simulink model "AGTF30SysDyn_PExPIn"  (R2023b)
settings: Solver=ode4  StartTime=0.0  StopTime=MWS.In.tend  FixedStep=MWS.In.Ts  RelTol=1e-3  EnableMultiTasking=on
model workspace: external: MAT-File (data not in the file)
values from neighbouring files (symbols this model uses):
  MWS = setup_initialize(MWS,startPt,SSsolverSP)    [Setup_Simulation.m]    (also in run_AGTF30e_script.m = Setup_Simulation(inputMethod,MWS.In,filename,Mdl,SSsolverSP))
undefined symbols (not defined in the file or in its folder): DiscIntNeverNeededParam
libraries: simulink x32, Lib_Solve_ModelSource_TMATS x28, Lib_EMTAT x27, Lib_Cntrl_FirstOrderSensor_TMATS x19, Lib_Cntrl_FirstOrderActuator_TMATS x2, Lib_Cntrl_LimitSelect_TMATS x2, Lib_Solve_OuterLoopIntegrator_TMATS x2, Lib_Cntrl_CorrectedSpeed_TMATS x1, Lib_Solve_IterNRSolverJC_TMATS x1, slpidlib x1
(part 1 of 8)
settings Model: Creator=jwchapm2  LastModifiedBy=jlkratz
settings SolverCC: AlgebraicLoopSolver=TrustRegion
settings DataIOCC: LimitDataPoints=on  SaveFormat=Array  ReturnWorkspaceOutputs=off
settings OptimizationCC: LifeSpan=inf
settings DebuggingCC: UnconnectedInputMsg=warning  UnconnectedOutputMsg=warning  UnconnectedLineMsg=warning  SFUnexpectedBacktrackingDiag=warning  SFNoUnconditionalDefaultTransitionDiag=warning  SFExecutionAtInitializationDiag=none  ArithmeticOperatorsInVariantConditions=warning
settings HardwareCC: ProdBitPerPointer=32  ProdBitPerSizeT=32  ProdBitPerPtrDiffT=32  ProdLargestAtomicFloat=None  ProdIntDivRoundTo=Undefined  ProdEndianess=Unspecified  ProdWordSize=32  ProdHWDeviceType=32-bit Generic
settings ModelReferenceCC: EnableRefExpFcnMdlSchedulingChecks=on  PropagateSignalLabelsOutOfModel=off
settings SFSimCC: SimUseLocalCustomCode=off  CustomCodeUndefinedFunction=UseInterfaceOnly
settings RTWCC: RTWUseLocalCustomCode=off  DLArmComputeVersion=19.05
settings CodeAppCC: StateflowObjectComments=on
settings GRTTargetCC: TargetLangStandard=C89/C90 (ANSI)
settings ConfigComp: CovMetricSettings=dw  CovSaveCumulativeToWorkspaceVar=on  CovSaveSingleToWorkspaceVar=on  CovExternalEMLEnable=off

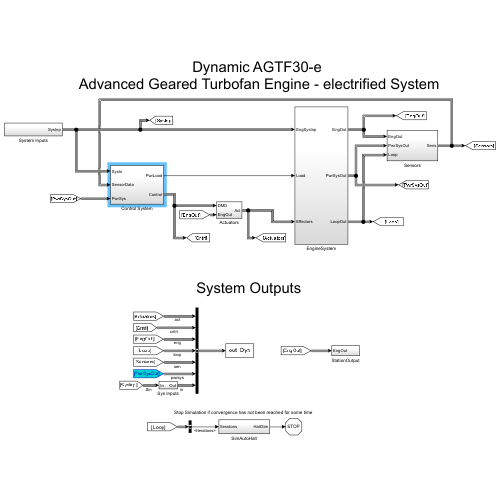
[thumbnail: Simulink's stored preview of the top-level diagram]
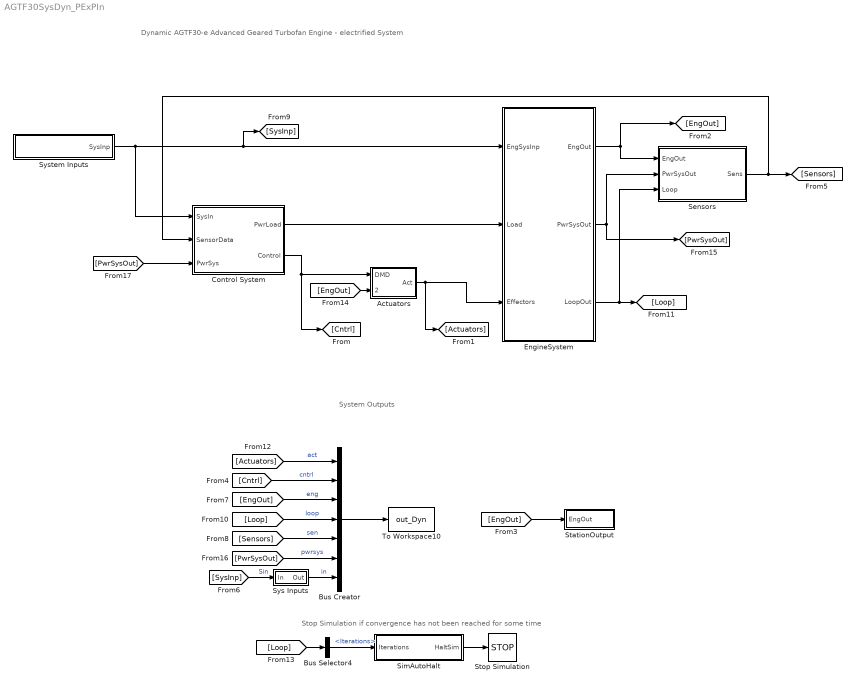
== system AGTF30SysDyn_PExPIn ==
  note: Stop Simulation if convergence has not been reached for some time
  note: Dynamic AGTF30-e
      | Advanced Geared Turbofan Engine - electrified System
  note: System Outputs
  Actuators : Subsystem
  Bus Creator : BusCreator  Inputs=7
  Bus Selector4 : BusSelector  OutputSignals=Solver.Iterations
  Control System : Subsystem
  EngineSystem : Subsystem
  Sensors : Subsystem
  SimAutoHalt : Subsystem
  StationOutput : Subsystem
  Stop Simulation : Stop
  Sys Inputs : Subsystem
  System Inputs : Subsystem
  To Workspace10 : ToWorkspace  VariableName=out_Dyn  SaveFormat=Timeseries  SampleTime=-1
  wires:
  Actuators/1(Act) -> [Actuators], EngineSystem/3(Effectors)
  Control System/2(Control) -> [Cntrl], Actuators/1(DMD)
  System Inputs/1(SysInp) -> Control System/1(SysIn), EngineSystem/1(EngSysInp), [SysInp]
  EngineSystem/1(EngOut) -> Sensors/1(EngOut), [EngOut]
  EngineSystem/3(LoopOut) -> Sensors/3(Loop), [Loop]
  [EngOut] -> StationOutput/1(EngOut)
  Bus Creator/1 -> To Workspace10/1
  [Loop] -> Bus Creator/4  "loop"
  [Sensors] -> Bus Creator/5  "sen"
  [EngOut] -> Bus Creator/3  "eng"
  Sys Inputs/1(Out) -> Bus Creator/7  "in"
  [Actuators] -> Bus Creator/1  "act"
  [Cntrl] -> Bus Creator/2  "cntrl"
  Sensors/1(Sens) -> Control System/2(SensorData), [Sensors]
  [Loop] -> Bus Selector4/1
  Bus Selector4/1 -> SimAutoHalt/1(Iterations)  "<Iterations>"
  SimAutoHalt/1(HaltSim) -> Stop Simulation/1
  [SysInp] -> Sys Inputs/1(In)  "Sin"
  EngineSystem/2(PwrSysOut) -> Sensors/2(PwrSysOut), [PwrSysOut]
  Control System/1(PwrLoad) -> EngineSystem/2(Load)
  [EngOut] -> Actuators/2(EngOut)
  [PwrSysOut] -> Bus Creator/6  "pwrsys"
  [PwrSysOut] -> Control System/3(PwrSys)

== system AGTF30SysDyn_PExPIn/Actuators ==
  DMD : Inport
  EngOut : Inport  Port=2
  Bus Creator : BusCreator  Inputs=9
  Bus Selector : BusSelector  OutputSignals=GBData.DEM.Nem,GBData.PGB.Nem
  Bus Selector1 : BusSelector  OutputSignals=Dmd.Wfdmd,Dmd.VBVdmd,Dmd.VAFNdmd,Dmd.TrqEMLdmd,Dmd.TrqEMHdmd,Dmd.TrqEMSdmd,Dmd.TrqEMRdmd,Dmd.TrqEMCdmd,Dmd.TrqEMPdmd
  Carrier Electric Machine : Subsystem
  Demux : Demux  Outputs=2
  Demux1 : Demux
  FMV : Subsystem
  HPS Electric Machine : Subsystem
  LPS Electric Machine : Subsystem
  Planet Gear Electric Machine : Subsystem
  Ring Gear Electric Machine : Subsystem
  Sun Gear Electric Machine : Subsystem
  VAFN : Subsystem
  VBV : Subsystem
  Act : Outport
  wires:
  DMD/1 -> Bus Selector1/1
  Bus Creator/1 -> Act/1  "Actuator"
  Bus Selector1/3 -> VAFN/1(VAFNdmd)  "<VAFNdmd>"
  Bus Selector1/2 -> VBV/1(VBVdmd)  "<VBVdmd>"
  VBV/1(VBVact) -> Bus Creator/2  "VBVact"
  VAFN/1(VAFNact) -> Bus Creator/3  "VAFNact"
  Bus Selector1/1 -> FMV/1(Wfdmd)  "<Wfdmd>"
  FMV/1(Wfact) -> Bus Creator/1  "Wfact"
  LPS Electric Machine/1(TrqEMLact) -> Bus Creator/4  "TrqEML"
  HPS Electric Machine/1(TrqEMHact) -> Bus Creator/5  "TrqEMH"
  Sun Gear Electric Machine/1(TrqEMSact) -> Bus Creator/6  "TrqEMS"
  Ring Gear Electric Machine/1(TrqEMRact) -> Bus Creator/7  "TrqEMR"
  Carrier Electric Machine/1(TrqEMCact) -> Bus Creator/8  "TrqEMC"
  Planet Gear Electric Machine/1(TrqEMPact) -> Bus Creator/9  "TrqEMP"
  Bus Selector1/4 -> LPS Electric Machine/1(TrqEMLdmd)  "<TrqEMLdmd>"
  Bus Selector1/5 -> HPS Electric Machine/1(TrqEMHdmd)  "<TrqEMHdmd>"
  Bus Selector1/6 -> Sun Gear Electric Machine/1(TrqEMSdmd)  "<TrqEMSdmd>"
  Bus Selector1/7 -> Ring Gear Electric Machine/1(TrqEMRdmd)  "<TrqEMRdmd>"
  Bus Selector1/8 -> Carrier Electric Machine/1(TrqEMCdmd)  "<TrqEMCdmd>"
  Bus Selector1/9 -> Planet Gear Electric Machine/1(TrqEMPdmd)  "<TrqEMPdmd>"
  EngOut/1 -> Bus Selector/1
  Bus Selector/1 -> Demux/1  "<Nem>"
  Bus Selector/2 -> Demux1/1  "<Nem>"
  Demux/1 -> LPS Electric Machine/2(NemL)
  Demux/2 -> HPS Electric Machine/2(NemH)
  Demux1/1 -> Sun Gear Electric Machine/2(NemS)
  Demux1/2 -> Ring Gear Electric Machine/2(NemR)
  Demux1/3 -> Carrier Electric Machine/2(NemC)
  Demux1/4 -> Planet Gear Electric Machine/2(NemP)

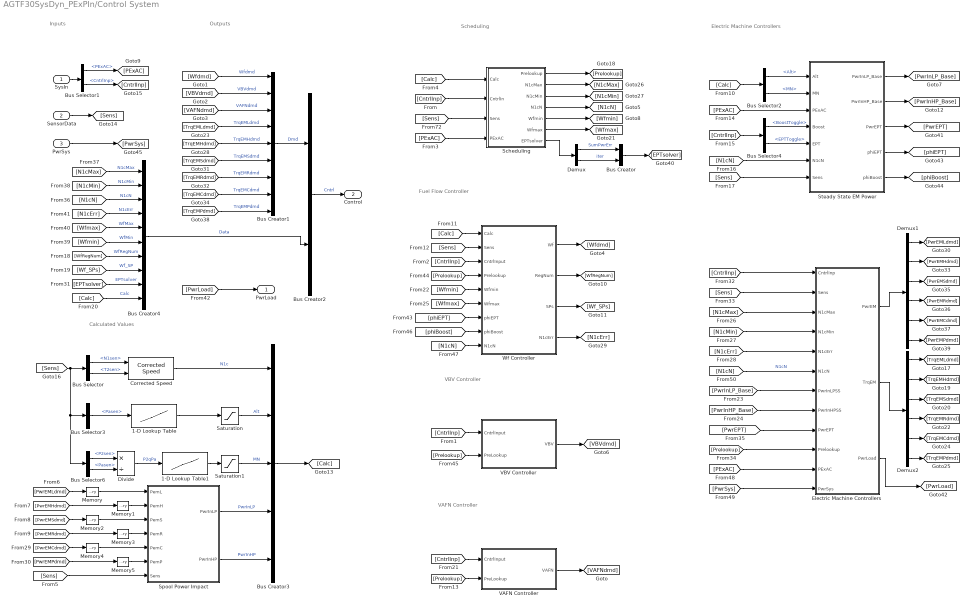
== system AGTF30SysDyn_PExPIn/Control System ==
  note: Inputs
  note: Calculated Values
  note: Outputs
  note: Fuel Flow Controller
  note: VBV Controller
  note: Scheduling
  note: VAFN Controller
  note: Electric Machine Controllers
  SysIn : Inport
  SensorData : Inport  Port=2
  PwrSys : Inport  Port=3
  1-D Lookup Table : Lookup_n-D  NumberOfTableDimensions=1  BreakpointsForDimension1=MWS.Cntrl.AltCalc_PaVec  Table=MWS.Cntrl.AltCalc_AltVec  InternalRulePriority=Speed  RndMeth=Simplest
  1-D Lookup Table1 : Lookup_n-D  NumberOfTableDimensions=1  BreakpointsForDimension1=MWS.Cntrl.MNCalc_P2qPa  Table=MWS.Cntrl.MNCalc_MNVec  InternalRulePriority=Speed  RndMeth=Simplest
  Bus Creator : BusCreator  Inputs=2
  Bus Creator1 : BusCreator  Inputs=9
  Bus Creator2 : BusCreator  Inputs=2
  Bus Creator3 : BusCreator  Inputs=5
  Bus Creator4 : BusCreator  Inputs=10
  Bus Selector : BusSelector  OutputSignals=N.N1sen,T.T2sen
  Bus Selector1 : BusSelector  OutputSignals=EngInp.PExAC,CntrlInp
  Bus Selector2 : BusSelector  OutputSignals=Alt,MN
  Bus Selector3 : BusSelector  OutputSignals=P.Pasen
  Bus Selector4 : BusSelector  OutputSignals=PilotCmd.BoostToggle,PilotCmd.EPTToggle
  Bus Selector6 : BusSelector  OutputSignals=P.P2sen,P.Pasen
  Corrected Speed : Lib_Cntrl_CorrectedSpeed_TMATS/Corrected Speed  C_TSTD_M=518.67
  Demux : Demux  Outputs=2
  Demux1 : Demux  Outputs=6
  Demux2 : Demux  Outputs=6
  Divide : Product  Inputs=*/
  Electric Machine Controllers : Subsystem
  Memory : Memory  InitialCondition=MWS.Init.IC.PwrEML
  Memory1 : Memory  InitialCondition=MWS.Init.IC.PwrEMH
  Memory2 : Memory  InitialCondition=MWS.Init.IC.PwrEMS
  Memory3 : Memory  InitialCondition=MWS.Init.IC.PwrEMR
  Memory4 : Memory  InitialCondition=MWS.Init.IC.PwrEMC
  Memory5 : Memory  InitialCondition=MWS.Init.IC.PwrEMP
  Saturation : Saturate  UpperLimit=MWS.Cntrl.AltCalc_Altmax  LowerLimit=MWS.Cntrl.AltCalc_Altmin
  Saturation1 : Saturate  UpperLimit=MWS.Cntrl.MNCalc_MNmax  LowerLimit=MWS.Cntrl.MNCalc_MNmin
  Scheduling : Subsystem
  Spool Power Impact : Subsystem
  Steady State EM Power : Subsystem
  VAFN Controller : Subsystem
  VBV Controller : Subsystem
  Wf Controller : Subsystem
  PwrLoad : Outport
  Control : Outport  Port=2
  wires:
  [Wfdmd] -> Bus Creator1/1  "Wfdmd"
  [VBVdmd] -> Bus Creator1/2  "VBVdmd"
  [VAFNdmd] -> Bus Creator1/3  "VAFNdmd"
  SensorData/1 -> [Sens]
  Bus Selector/1 -> Corrected Speed/1  "<N1sen>"
  Corrected Speed/1 -> Bus Creator3/1  "N1c"
  Bus Selector/2 -> Corrected Speed/2  "<T2sen>"
  1-D Lookup Table/1 -> Saturation/1
  [Sens] -> Bus Selector6/1, Bus Selector3/1, Bus Selector/1
  Bus Selector3/1 -> 1-D Lookup Table/1  "<Pasen>"
  Bus Selector6/1 -> Divide/1  "<P2sen>"
  Bus Selector6/2 -> Divide/2  "<Pasen>"
  Divide/1 -> 1-D Lookup Table1/1  "P2qPa"
  1-D Lookup Table1/1 -> Saturation1/1
  Saturation/1 -> Bus Creator3/2  "Alt"
  Saturation1/1 -> Bus Creator3/3  "MN"
  Bus Creator2/1 -> Control/1  "Cntrl"
  [TrqEMLdmd] -> Bus Creator1/4  "TrqEMLdmd"
  [TrqEMHdmd] -> Bus Creator1/5  "TrqEMHdmd"
  [TrqEMSdmd] -> Bus Creator1/6  "TrqEMSdmd"
  [TrqEMRdmd] -> Bus Creator1/7  "TrqEMRdmd"
  [TrqEMCdmd] -> Bus Creator1/8  "TrqEMCdmd"
  [TrqEMPdmd] -> Bus Creator1/9  "TrqEMPdmd"
  Bus Creator1/1 -> Bus Creator2/1  "Dmd"
  [Wfmax] -> Wf Controller/6(Wfmax)
  [Calc] -> Wf Controller/1(Calc)
  [Wfmin] -> Wf Controller/5(Wfmin)
  [Sens] -> Wf Controller/2(Sens)
  Wf Controller/1(Wf) -> [Wfdmd]
  [CntrlInp] -> Wf Controller/3(CntrlInput)
  Wf Controller/2(RegNum) -> [WfRegNum]
  Wf Controller/3(SPs) -> [Wf_SPs]
  [Prelookup] -> Wf Controller/4(Prelookup)
  [Prelookup] -> VBV Controller/2(PreLookup)
  VBV Controller/1(VBV) -> [VBVdmd]
  Scheduling/5(Wfmin) -> [Wfmin]
  Scheduling/4(N1cN) -> [N1cN]
  Scheduling/6(Wfmax) -> [Wfmax]
  Scheduling/1(Prelookup) -> [Prelookup]
  [CntrlInp] -> Scheduling/2(CntrlIn)
  [Sens] -> Scheduling/3(Sens)
  [Prelookup] -> VAFN Controller/2(PreLookup)
  VAFN Controller/1(VAFN) -> [VAFNdmd]
  SysIn/1 -> Bus Selector1/1
  Bus Selector1/2 -> [CntrlInp]  "<CntrlInp>"
  Bus Selector1/1 -> [PExAC]  "<PExAC>"
  Bus Creator3/1 -> [Calc]
  [Calc] -> Scheduling/1(Calc)
  Spool Power Impact/1(PwrInLP) -> Bus Creator3/4  "PwrInLP"
  Spool Power Impact/2(PwrInHP) -> Bus Creator3/5  "PwrInHP"
  [PExAC] -> Scheduling/4(PExAC)
  [PwrEMSdmd] -> Memory2/1
  [PwrEMRdmd] -> Memory3/1
  [PwrEMCdmd] -> Memory4/1
  [PwrEMPdmd] -> Memory5/1
  [PwrEMHdmd] -> Memory1/1
  [PwrEMLdmd] -> Memory/1
  [Sens] -> Spool Power Impact/7(Sens)
  Memory/1 -> Spool Power Impact/1(PemL)
  Memory1/1 -> Spool Power Impact/2(PemH)
  Memory2/1 -> Spool Power Impact/3(PemS)
  Memory3/1 -> Spool Power Impact/4(PemR)
  Memory4/1 -> Spool Power Impact/5(PemC)
  Memory5/1 -> Spool Power Impact/6(PemP)
  [CntrlInp] -> VAFN Controller/1(CntrlInput)
  [CntrlInp] -> VBV Controller/1(CntrlInput)
  Steady State EM Power/1(PwrInLP_Base) -> [PwrInLP_Base]
  Steady State EM Power/2(PwrInHP_Base) -> [PwrInHP_Base]
  [Calc] -> Bus Selector2/1
  Bus Selector2/1 -> Steady State EM Power/1(Alt)  "<Alt>"
  Bus Selector2/2 -> Steady State EM Power/2(MN)  "<MN>"
  [PExAC] -> Steady State EM Power/3(PExAC)
  [CntrlInp] -> Bus Selector4/1
  Bus Selector4/1 -> Steady State EM Power/4(Boost)  "<BoostToggle>"
  Bus Selector4/2 -> Steady State EM Power/5(EPT)  "<EPTToggle>"
  [N1cN] -> Steady State EM Power/6(N1cN)
  [Sens] -> Steady State EM Power/7(Sens)
  Scheduling/2(N1cMax) -> [N1cMax]
  Scheduling/3(N1cMin) -> [N1cMin]
  Wf Controller/4(N1cErr) -> [N1cErr]
  Scheduling/7(EPTsolver) -> Demux/1
  Demux/1 -> Bus Creator/1  "SumPwrErr"
  Demux/2 -> Bus Creator/2  "iter"
  Bus Creator/1 -> [EPTsolver]
  [PwrInHP_Base] -> Electric Machine Controllers/8(PwrInHPSS)
  [CntrlInp] -> Electric Machine Controllers/1(CntrlInp)
  [PwrInLP_Base] -> Electric Machine Controllers/7(PwrInLPSS)
  [N1cMax] -> Electric Machine Controllers/3(N1cMax)
  [N1cMin] -> Electric Machine Controllers/4(N1cMin)
  [N1cErr] -> Electric Machine Controllers/5(N1cErr)
  Demux1/1 -> [PwrEMLdmd]
  Demux1/2 -> [PwrEMHdmd]
  Demux1/3 -> [PwrEMSdmd]
  Demux1/4 -> [PwrEMRdmd]
  Demux1/5 -> [PwrEMCdmd]
  Demux1/6 -> [PwrEMPdmd]
  Demux2/1 -> [TrqEMLdmd]
  Demux2/2 -> [TrqEMHdmd]
  Demux2/3 -> [TrqEMSdmd]
  Demux2/4 -> [TrqEMRdmd]
  Demux2/5 -> [TrqEMCdmd]
  Demux2/6 -> [TrqEMPdmd]
  [Sens] -> Electric Machine Controllers/2(Sens)
  [Prelookup] -> Electric Machine Controllers/10(Prelookup)
  Electric Machine Controllers/1(PwrEM) -> Demux1/1
  Electric Machine Controllers/2(TrqEM) -> Demux2/1
  Steady State EM Power/3(PwrEPT) -> [PwrEPT]
  [PwrEPT] -> Electric Machine Controllers/9(PwrEPT)
  [EPTsolver] -> Bus Creator4/9  "EPTsolver"
  [Wf_SPs] -> Bus Creator4/8  "Wf_SP"
  [WfRegNum] -> Bus Creator4/7  "WfRegNum"
  [Wfmin] -> Bus Creator4/6  "WfMin"
  [Wfmax] -> Bus Creator4/5  "WfMax"
  [N1cErr] -> Bus Creator4/4  "N1cErr"
  [N1cN] -> Bus Creator4/3  "N1cN"
  [N1cMin] -> Bus Creator4/2  "N1cMin"
  [N1cMax] -> Bus Creator4/1  "N1cMax"
  [Calc] -> Bus Creator4/10  "Calc"
  Bus Creator4/1 -> Bus Creator2/2  "Data"
  [PwrLoad] -> PwrLoad/1
  Steady State EM Power/4(phiEPT) -> [phiEPT]
  Steady State EM Power/5(phiBoost) -> [phiBoost]
  [phiEPT] -> Wf Controller/7(phiEPT)
  [phiBoost] -> Wf Controller/8(phiBoost)
  [N1cN] -> Wf Controller/9(N1cN)
  [PwrSys] -> Electric Machine Controllers/12(PwrSys)
  PwrSys/1 -> [PwrSys]
  Electric Machine Controllers/3(PwrLoad) -> [PwrLoad]
  [PExAC] -> Electric Machine Controllers/11(PExAC)
  [N1cN] -> Electric Machine Controllers/6(N1cN)  "N1cN"

== system AGTF30SysDyn_PExPIn/EngineSystem ==
  note: Shaft Integrators
  note: Engine State
      | Integration Loop
  note: Engine Data Output
  note: Power System Data Output
  EngSysInp : Inport
  Load : Inport  Port=2
  Effectors : Inport  Port=3
  Bus Creator : BusCreator  Inputs=5
  EngineDW : Subsystem
  HP speed integrator : Lib_Solve_OuterLoopIntegrator_TMATS/OuterLoop integrator  OL_IC_M=MWS.Init.IC.N3
  LP shaft speed integrator : Lib_Solve_OuterLoopIntegrator_TMATS/OuterLoop integrator  OL_IC_M=MWS.Init.IC.N2
  Power System : Subsystem
  EngOut : Outport
  PwrSysOut : Outport  Port=2
  LoopOut : Outport  Port=3
  wires:
  EngSysInp/1 -> EngineDW/1(EngSysInp)
  LP shaft speed integrator/1 -> [N2], EngineDW/3(N2)  "N2int"
  Effectors/1 -> Power System/3(TrqEM), EngineDW/2(Effectors)
  EngineDW/3(N2dot) -> LP shaft speed integrator/1, [N2dot]  "N2dot"
  EngineDW/2(Solver) -> Bus Creator/1  "Solver"
  EngineDW/1(EngOut) -> [EngOut], EngOut/1
  EngineDW/4(N3dot) -> HP speed integrator/1, [N3dot]  "N3dot"
  HP speed integrator/1 -> [N3], EngineDW/4(N3)  "N3int"
  Bus Creator/1 -> LoopOut/1  "Loop"
  [N3dot] -> Bus Creator/2
  [N2dot] -> Bus Creator/3
  [N2] -> Bus Creator/4
  [N3] -> Bus Creator/5
  [EngOut] -> Power System/2(Nem)
  Power System/1(PwrSysOut) -> PwrSysOut/1
  Load/1 -> Power System/1(Load [hp])

== system AGTF30SysDyn_PExPIn/Sensors ==
  note: Pressure Sensors
  note: Temperature Sensors
  note: Speed Sensors
  EngOut : Inport
  PwrSysOut : Inport  Port=2
  Loop : Inport  Port=3
  Bus Creator : BusCreator  Inputs=4
  Bus Creator1 : BusCreator  Inputs=4
  Bus Creator2 : BusCreator  Inputs=5
  Bus Creator3 : BusCreator  Inputs=9
  Bus Selector : BusSelector  OutputSignals=Amb.Pa,S2.Pt,S25.Pt,S36.Ps,S5.Pt
  Bus Selector1 : BusSelector  OutputSignals=S2.Tt,S36.Tt,S4.Tt,S45.Tt
  Bus Selector2 : BusSelector  OutputSignals=N2int,N3int
  Bus Selector3 : BusSelector  OutputSignals=GBData.DEM.Nem,GBData.PGB.Nem
  Bus Selector4 : BusSelector  OutputSignals=SOC
  Demux : Demux  Outputs=2
  Demux1 : Demux
  Gain : Gain  Gain=1/MWS.GearBox.GearRatio
  N1 sensor : Lib_Cntrl_FirstOrderSensor_TMATS/1st order  Sensor  IC_M=MWS.Init.IC.N1  Sen_Max_M=MWS.Sensor.N1.Max  Sen_Min_M=MWS.Sensor.N1.Min  Gain_M=1  Tau_M=MWS.Sensor.N1.Tau  GN_EN_M=off  GN_NST_M=MWS.In.Ts  GN_C_M=1  GN_MinNoise_M=0.3  F_Gain_M=1  F_Drift_M=0
  N2 sensor : Lib_Cntrl_FirstOrderSensor_TMATS/1st order  Sensor  IC_M=MWS.Init.IC.N2  Sen_Max_M=MWS.Sensor.N2.Max  Sen_Min_M=MWS.Sensor.N2.Min  Gain_M=1  Tau_M=MWS.Sensor.N2.Tau  GN_EN_M=off  GN_NST_M=MWS.In.Ts  GN_C_M=1  GN_MinNoise_M=0.3  F_Gain_M=1  F_Drift_M=0
  N3 sensor : Lib_Cntrl_FirstOrderSensor_TMATS/1st order  Sensor  IC_M=MWS.Init.IC.N3  Sen_Max_M=MWS.Sensor.N3.Max  Sen_Min_M=MWS.Sensor.N3.Min  Gain_M=1  Tau_M=MWS.Sensor.N3.Tau  GN_EN_M=off  GN_NST_M=MWS.In.Ts  GN_C_M=1  GN_MinNoise_M=0.3  F_Gain_M=1  F_Drift_M=0
  NemC sensor : Lib_Cntrl_FirstOrderSensor_TMATS/1st order  Sensor  IC_M=MWS.Init.IC.NemC  Sen_Max_M=MWS.Sensor.NemC.Max  Sen_Min_M=MWS.Sensor.NemC.Min  Gain_M=1  Tau_M=MWS.Sensor.NemC.Tau  GN_EN_M=off  GN_NST_M=MWS.In.Ts  GN_C_M=1  GN_MinNoise_M=0.3  F_Gain_M=1  F_Drift_M=0
  NemH sensor : Lib_Cntrl_FirstOrderSensor_TMATS/1st order  Sensor  IC_M=MWS.Init.IC.NemH  Sen_Max_M=MWS.Sensor.NemH.Max  Sen_Min_M=MWS.Sensor.NemH.Min  Gain_M=1  Tau_M=MWS.Sensor.NemH.Tau  GN_EN_M=off  GN_NST_M=MWS.In.Ts  GN_C_M=1  GN_MinNoise_M=0.3  F_Gain_M=1  F_Drift_M=0
  NemL sensor : Lib_Cntrl_FirstOrderSensor_TMATS/1st order  Sensor  IC_M=MWS.Init.IC.NemL  Sen_Max_M=MWS.Sensor.NemL.Max  Sen_Min_M=MWS.Sensor.NemL.Min  Gain_M=1  Tau_M=MWS.Sensor.NemL.Tau  GN_EN_M=off  GN_NST_M=MWS.In.Ts  GN_C_M=1  GN_MinNoise_M=0.3  F_Gain_M=1  F_Drift_M=0
  NemP sensor : Lib_Cntrl_FirstOrderSensor_TMATS/1st order  Sensor  IC_M=MWS.Init.IC.NemP  Sen_Max_M=MWS.Sensor.NemP.Max  Sen_Min_M=MWS.Sensor.NemP.Min  Gain_M=1  Tau_M=MWS.Sensor.NemP.Tau  GN_EN_M=off  GN_NST_M=MWS.In.Ts  GN_C_M=1  GN_MinNoise_M=0.3  F_Gain_M=1  F_Drift_M=0
  NemR sensor : Lib_Cntrl_FirstOrderSensor_TMATS/1st order  Sensor  IC_M=MWS.Init.IC.NemR  Sen_Max_M=MWS.Sensor.NemR.Max  Sen_Min_M=MWS.Sensor.NemR.Min  Gain_M=1  Tau_M=MWS.Sensor.NemR.Tau  GN_EN_M=off  GN_NST_M=MWS.In.Ts  GN_C_M=1  GN_MinNoise_M=0.3  F_Gain_M=1  F_Drift_M=0
  NemS sensor : Lib_Cntrl_FirstOrderSensor_TMATS/1st order  Sensor  IC_M=MWS.Init.IC.NemS  Sen_Max_M=MWS.Sensor.NemS.Max  Sen_Min_M=MWS.Sensor.NemS.Min  Gain_M=1  Tau_M=MWS.Sensor.NemS.Tau  GN_EN_M=off  GN_NST_M=MWS.In.Ts  GN_C_M=1  GN_MinNoise_M=0.3  F_Gain_M=1  F_Drift_M=0
  Pamb sensor : Lib_Cntrl_FirstOrderSensor_TMATS/1st order  Sensor  IC_M=MWS.Init.IC.Pa  Sen_Max_M=MWS.Sensor.P2.Max  Sen_Min_M=MWS.Sensor.P2.Min  Gain_M=1  Tau_M=MWS.Sensor.P2.Tau  GN_EN_M=off  GN_NST_M=MWS.In.Ts  GN_C_M=1  GN_MinNoise_M=0.3  F_Gain_M=1  F_Drift_M=0
  Ps3 sensor : Lib_Cntrl_FirstOrderSensor_TMATS/1st order  Sensor  IC_M=MWS.Init.IC.Ps3  Sen_Max_M=MWS.Sensor.Ps3.Max  Sen_Min_M=MWS.Sensor.Ps3.Min  Gain_M=1  Tau_M=MWS.Sensor.Ps3.Tau  GN_EN_M=off  GN_NST_M=MWS.In.Ts  GN_C_M=1  GN_MinNoise_M=0.3  F_Gain_M=1  F_Drift_M=0
  Pt2 sensor : Lib_Cntrl_FirstOrderSensor_TMATS/1st order  Sensor  IC_M=MWS.Init.IC.P2  Sen_Max_M=MWS.Sensor.P2.Max  Sen_Min_M=MWS.Sensor.P2.Min  Gain_M=1  Tau_M=MWS.Sensor.P2.Tau  GN_EN_M=off  GN_NST_M=MWS.In.Ts  GN_C_M=1  GN_MinNoise_M=0.3  F_Gain_M=1  F_Drift_M=0
  Pt25 sensor : Lib_Cntrl_FirstOrderSensor_TMATS/1st order  Sensor  IC_M=MWS.Init.IC.P25  Sen_Max_M=MWS.Sensor.P25.Max  Sen_Min_M=MWS.Sensor.P25.Min  Gain_M=1  Tau_M=MWS.Sensor.P25.Tau  GN_EN_M=off  GN_NST_M=MWS.In.Ts  GN_C_M=1  GN_MinNoise_M=0.3  F_Gain_M=1  F_Drift_M=0
  Pt5 sensor : Lib_Cntrl_FirstOrderSensor_TMATS/1st order  Sensor  IC_M=MWS.Init.IC.P5  Sen_Max_M=MWS.Sensor.P5.Max  Sen_Min_M=MWS.Sensor.P5.Min  Gain_M=1  Tau_M=MWS.Sensor.P5.Tau  GN_EN_M=off  GN_NST_M=MWS.In.Ts  GN_C_M=1  GN_MinNoise_M=0.3  F_Gain_M=1  F_Drift_M=0
  SOC sensor : Lib_Cntrl_FirstOrderSensor_TMATS/1st order  Sensor  IC_M=MWS.Init.IC.SOC  Sen_Max_M=MWS.Sensor.SOC.Max  Sen_Min_M=MWS.Sensor.SOC.Min  Gain_M=1  Tau_M=MWS.Sensor.SOC.Tau  GN_EN_M=off  GN_NST_M=MWS.In.Ts  GN_C_M=1  GN_MinNoise_M=0.3  F_Gain_M=1  F_Drift_M=0
  T2 sensor : Lib_Cntrl_FirstOrderSensor_TMATS/1st order  Sensor  IC_M=MWS.Init.IC.T2  Sen_Max_M=MWS.Sensor.T2.Max  Sen_Min_M=MWS.Sensor.T2.Min  Gain_M=1  Tau_M=MWS.Sensor.T2.Tau  GN_EN_M=off  GN_NST_M=MWS.In.Ts  GN_C_M=1  GN_MinNoise_M=0.3  F_Gain_M=1  F_Drift_M=0
  T3 sensor : Lib_Cntrl_FirstOrderSensor_TMATS/1st order  Sensor  IC_M=MWS.Init.IC.T3  Sen_Max_M=MWS.Sensor.T3.Max  Sen_Min_M=MWS.Sensor.T3.Min  Gain_M=1  Tau_M=MWS.Sensor.T3.Tau  GN_EN_M=off  GN_NST_M=MWS.In.Ts  GN_C_M=1  GN_MinNoise_M=0.3  F_Gain_M=1  F_Drift_M=0
  T4 sensor : Lib_Cntrl_FirstOrderSensor_TMATS/1st order  Sensor  IC_M=MWS.Init.IC.T4  Sen_Max_M=MWS.Sensor.T4.Max  Sen_Min_M=MWS.Sensor.T4.Min  Gain_M=1  Tau_M=MWS.Sensor.T4.Tau  GN_EN_M=off  GN_NST_M=MWS.In.Ts  GN_C_M=1  GN_MinNoise_M=0.3  F_Gain_M=1  F_Drift_M=0
  T45 sensor : Lib_Cntrl_FirstOrderSensor_TMATS/1st order  Sensor  IC_M=MWS.Init.IC.T45  Sen_Max_M=MWS.Sensor.T45.Max  Sen_Min_M=MWS.Sensor.T45.Min  Gain_M=1  Tau_M=MWS.Sensor.T45.Tau  GN_EN_M=off  GN_NST_M=MWS.In.Ts  GN_C_M=1  GN_MinNoise_M=0.3  F_Gain_M=1  F_Drift_M=0
  Sens : Outport
  wires:
  Bus Creator/1 -> Sens/1  "Sensors"
  Bus Selector/2 -> Pt2 sensor/1  "<Pt>"
  Bus Creator2/1 -> Bus Creator/1  "P"
  Bus Creator1/1 -> Bus Creator/2  "T"
  Bus Selector1/1 -> T2 sensor/1  "<Tt>"
  Bus Creator3/1 -> Bus Creator/3  "N"
  Bus Selector/3 -> Pt25 sensor/1  "<Pt>"
  Bus Selector/5 -> Pt5 sensor/1  "<Pt>"
  Pt2 sensor/1 -> Bus Creator2/2  "P2sen"
  Pt25 sensor/1 -> Bus Creator2/3  "P25sen"
  Pt5 sensor/1 -> Bus Creator2/5  "P5sen"
  Bus Selector1/2 -> T3 sensor/1  "<Tt>"
  Bus Selector1/4 -> T45 sensor/1  "<Tt>"
  T2 sensor/1 -> Bus Creator1/1  "T2sen"
  T3 sensor/1 -> Bus Creator1/2  "T3sen"
  N1 sensor/1 -> Bus Creator3/1  "N1sen"
  Bus Selector/4 -> Ps3 sensor/1  "<Ps>"
  N3 sensor/1 -> Bus Creator3/3  "N3sen"
  Bus Selector/1 -> Pamb sensor/1  "<Pa>"
  Pamb sensor/1 -> Bus Creator2/1  "Pasen"
  N2 sensor/1 -> Bus Creator3/2  "N2sen"
  EngOut/1 -> Bus Selector3/1, Bus Selector/1, Bus Selector1/1
  Bus Selector2/2 -> N3 sensor/1  "<N3int>"
  Bus Selector2/1 -> N2 sensor/1, Gain/1  "<N2int>"
  Gain/1 -> N1 sensor/1
  Loop/1 -> Bus Selector2/1
  T45 sensor/1 -> Bus Creator1/4  "T45sen"
  Ps3 sensor/1 -> Bus Creator2/4  "Ps3sen"
  Bus Selector3/1 -> Demux/1  "<Nem>"
  Bus Selector3/2 -> Demux1/1  "<Nem>"
  NemL sensor/1 -> Bus Creator3/4  "NemLsen"
  NemH sensor/1 -> Bus Creator3/5  "NemHsen"
  Demux1/1 -> NemS sensor/1
  Demux1/2 -> NemR sensor/1
  Demux1/3 -> NemC sensor/1
  Demux1/4 -> NemP sensor/1
  Demux/1 -> NemL sensor/1
  Demux/2 -> NemH sensor/1
  NemS sensor/1 -> Bus Creator3/6  "NemSsen"
  NemR sensor/1 -> Bus Creator3/7  "NemRsen"
  NemC sensor/1 -> Bus Creator3/8  "NemCsen"
  NemP sensor/1 -> Bus Creator3/9  "NemPsen"
  Bus Selector1/3 -> T4 sensor/1  "<Tt>"
  T4 sensor/1 -> Bus Creator1/3  "T4sen"
  SOC sensor/1 -> Bus Creator/4  "SOC"
  PwrSysOut/1 -> Bus Selector4/1
  Bus Selector4/1 -> SOC sensor/1  "<SOC>"

== system AGTF30SysDyn_PExPIn/SimAutoHalt ==
  Iterations : Inport
  Compare To Constant : simulink/Logic and Bit Operations/Compare To Constant  relop=>=  const=MWS.Init.Max_IterDyn  OutDataTypeStr=boolean
  Compare To Constant1 : simulink/Logic and Bit Operations/Compare To Constant  relop=>=  const=MWS.Init.DynRunNonConv  OutDataTypeStr=boolean
  Constant : Constant
  Product : Product
  Sum : Sum  Inputs=|++
  Unit Delay : UnitDelay  SampleTime=-1  HasFrameUpgradeWarning=on
  HaltSim : Outport
  wires:
  Compare To Constant1/1 -> HaltSim/1
  Iterations/1 -> Compare To Constant/1
  Compare To Constant/1 -> Product/1
  Constant/1 -> Sum/1
  Sum/1 -> Unit Delay/1
  Unit Delay/1 -> Product/2
  Product/1 -> Sum/2, Compare To Constant1/1

== system AGTF30SysDyn_PExPIn/StationOutput ==
  EngOut : Inport
  Bus Selector1 : BusSelector  OutputSignals=Data.FAN_Data,Data.LPC_Data,Data.HPC_Data,Data.HPT_Data,Data.LPT_Data
  Bus Selector2 : BusSelector  OutputSignals=S0,S2,S21,S25,S36,S4,S45,S5,S17
  To Workspace : ToWorkspace  VariableName=out_S0  SaveFormat=Timeseries  SampleTime=-1
  To Workspace1 : ToWorkspace  VariableName=out_S2  SaveFormat=Timeseries  SampleTime=-1
  To Workspace10 : ToWorkspace  VariableName=out_HPCmp  SaveFormat=Timeseries  SampleTime=-1
  To Workspace11 : ToWorkspace  VariableName=out_HPTmp  SaveFormat=Timeseries  SampleTime=-1
  To Workspace12 : ToWorkspace  VariableName=out_LPTmp  SaveFormat=Timeseries  SampleTime=-1
  To Workspace13 : ToWorkspace  VariableName=out_S21  SaveFormat=Timeseries  SampleTime=-1
  To Workspace2 : ToWorkspace  VariableName=out_S25  SaveFormat=Timeseries  SampleTime=-1
  To Workspace3 : ToWorkspace  VariableName=out_S36  SaveFormat=Timeseries  SampleTime=-1
  To Workspace4 : ToWorkspace  VariableName=out_S4  SaveFormat=Timeseries  SampleTime=-1
  To Workspace5 : ToWorkspace  VariableName=out_S45  SaveFormat=Timeseries  SampleTime=-1
  To Workspace6 : ToWorkspace  VariableName=out_S5  SaveFormat=Timeseries  SampleTime=-1
  To Workspace7 : ToWorkspace  VariableName=out_S17  SaveFormat=Timeseries  SampleTime=-1
  To Workspace8 : ToWorkspace  VariableName=out_FANmp  SaveFormat=Timeseries  SampleTime=-1
  To Workspace9 : ToWorkspace  VariableName=out_LPCmp  SaveFormat=Timeseries  SampleTime=-1
  wires:
  Bus Selector2/3 -> To Workspace13/1  "<S21>"
  Bus Selector2/1 -> To Workspace/1  "<S0>"
  EngOut/1 -> Bus Selector1/1, Bus Selector2/1
  Bus Selector2/2 -> To Workspace1/1  "<S2>"
  Bus Selector2/4 -> To Workspace2/1  "<S25>"
  Bus Selector2/5 -> To Workspace3/1  "<S36>"
  Bus Selector2/6 -> To Workspace4/1  "<S4>"
  Bus Selector2/7 -> To Workspace5/1  "<S45>"
  Bus Selector2/8 -> To Workspace6/1  "<S5>"
  Bus Selector2/9 -> To Workspace7/1  "<S17>"
  Bus Selector1/1 -> To Workspace8/1  "<FAN_Data>"
  Bus Selector1/2 -> To Workspace9/1  "<LPC_Data>"
  Bus Selector1/3 -> To Workspace10/1  "<HPC_Data>"
  Bus Selector1/4 -> To Workspace11/1  "<HPT_Data>"
  Bus Selector1/5 -> To Workspace12/1  "<LPT_Data>"

== system AGTF30SysDyn_PExPIn/Sys Inputs ==
  In : Inport
  Bus Creator1 : BusCreator  Inputs=28
  Bus Selector : BusSelector  OutputSignals=EngInp.Alt,EngInp.dT,EngInp.MN,EngInp.PExAC,CntrlInp.PilotCmd.PLA,CntrlInp.PilotCmd.BoostToggle,CntrlInp.PilotCmd.EPTToggle,CntrlInp.PilotCmd.ChargingToggle,CntrlInp.ManualOp.N1cMan,CntrlInp.ManualOp.WfMan,CntrlInp.ManualOp.VBVMan,CntrlInp.ManualOp.VAFNMan,CntrlInp.ManualOp.PwrInLPNomMan,CntrlInp.ManualOp.PwrInLPOffNomMan,CntrlInp.ManualOp.PwrInHPNomMan,CntrlInp.ManualOp.PwrInHPOffNomMan,CntrlInp.ManualOp.PwrInLPEMNomMan,CntrlInp.ManualOp.PwrInLPEMOffNomMan,CntrlInp.ManualOp.PwrInHPEMNomMan,CntrlInp.ManualOp.PwrInHPEMOffNomMan,CntrlInp.ManualOp.PwrInSEMNomMan,CntrlInp.ManualOp.PwrInSEMOffNomMan,CntrlInp.ManualOp.PwrInREMNomMan,CntrlInp.ManualOp.PwrInREMOffNomMan,CntrlInp.ManualOp.PwrInCEMNomMan,CntrlInp.ManualOp.PwrInCEMOffNomMan,CntrlInp.ManualOp.PwrInPEMNomMan,CntrlInp.ManualOp.PwrInPEMOffNomMan
  Out : Outport
  wires:
  In/1 -> Bus Selector/1
  Bus Selector/4 -> Bus Creator1/4  "<PExAC>"
  Bus Selector/6 -> Bus Creator1/6  "<BoostToggle>"
  Bus Selector/7 -> Bus Creator1/7  "<EPTToggle>"
  Bus Selector/8 -> Bus Creator1/8  "<ChargingToggle>"
  Bus Selector/10 -> Bus Creator1/10  "<WfMan>"
  Bus Selector/13 -> Bus Creator1/13  "<PwrInLPNomMan>"
  Bus Selector/3 -> Bus Creator1/3  "<MN>"
  Bus Selector/5 -> Bus Creator1/5  "<PLA>"
  Bus Selector/1 -> Bus Creator1/1  "<Alt>"
  Bus Selector/12 -> Bus Creator1/12  "<VAFNMan>"
  Bus Selector/2 -> Bus Creator1/2  "<dT>"
  Bus Creator1/1 -> Out/1
  Bus Selector/14 -> Bus Creator1/14  "<PwrInLPOffNomMan>"
  Bus Selector/15 -> Bus Creator1/15  "<PwrInHPNomMan>"
  Bus Selector/16 -> Bus Creator1/16  "<PwrInHPOffNomMan>"
  Bus Selector/17 -> Bus Creator1/17  "<PwrInLPEMNomMan>"
  Bus Selector/18 -> Bus Creator1/18  "<PwrInLPEMOffNomMan>"
  Bus Selector/19 -> Bus Creator1/19  "<PwrInHPEMNomMan>"
  Bus Selector/20 -> Bus Creator1/20  "<PwrInHPEMOffNomMan>"
  Bus Selector/22 -> Bus Creator1/22  "<PwrInSEMOffNomMan>"
  Bus Selector/23 -> Bus Creator1/23  "<PwrInREMNomMan>"
  Bus Selector/24 -> Bus Creator1/24  "<PwrInREMOffNomMan>"
  Bus Selector/26 -> Bus Creator1/26  "<PwrInCEMOffNomMan>"
  Bus Selector/27 -> Bus Creator1/27  "<PwrInPEMNomMan>"
  Bus Selector/28 -> Bus Creator1/28  "<PwrInPEMOffNomMan>"
  Bus Selector/25 -> Bus Creator1/25  "<PwrInCEMNomMan>"
  Bus Selector/21 -> Bus Creator1/21  "<PwrInSEMNomMan>"
  Bus Selector/11 -> Bus Creator1/11  "<VBVMan>"
  Bus Selector/9 -> Bus Creator1/9  "<N1cMan>"

== system AGTF30SysDyn_PExPIn/System Inputs ==
  note: Engine Inputs
  note: Control System Inputs
  note: 40 - 80 angle
  Bus Creator : BusCreator  Inputs=4
  Bus Creator1 : BusCreator  Inputs=4
  Bus Creator2 : BusCreator  Inputs=2
  Bus Creator5 : BusCreator  Inputs=2
  Bus Creator6 : BusCreator  Inputs=40
  Constant1 : Constant  Value=MWS.In.WfManEn
  Constant10 : Constant  Value=MWS.In.PwrInHPEMOffNomManEn
  Constant11 : Constant  Value=MWS.In.PwrInLPEMOffNomManEn
  Constant12 : Constant  Value=MWS.In.PwrInLPEMNomManEn
  Constant13 : Constant  Value=MWS.In.PwrInSEMOffNomManEn
  Constant14 : Constant  Value=MWS.In.PwrInSEMNomManEn
  Constant15 : Constant  Value=MWS.In.PwrInREMOffNomManEn
  Constant16 : Constant  Value=MWS.In.PwrInREMNomManEn
  Constant17 : Constant  Value=MWS.In.PwrInCEMOffNomManEn
  Constant18 : Constant  Value=MWS.In.PwrInCEMNomManEn
  Constant19 : Constant  Value=MWS.In.PwrInPEMOffNomManEn
  Constant2 : Constant  Value=MWS.In.PwrInLPNomManEn
  Constant20 : Constant  Value=MWS.In.PwrInPEMNomManEn
  Constant3 : Constant  Value=MWS.In.VBVManEn
  Constant4 : Constant  Value=MWS.In.VAFNManEn
  Constant5 : Constant  Value=MWS.In.N1cManEn
  Constant6 : Constant  Value=MWS.In.PwrInHPNomManEn
  Constant7 : Constant  Value=MWS.In.PwrInLPOffNomManEn
  Constant8 : Constant  Value=MWS.In.PwrInHPOffNomManEn
  Constant9 : Constant  Value=MWS.In.PwrInHPEMNomManEn
  Model Source : Lib_Solve_ModelSource_TMATS/Model Source  T_vec_M=MWS.In.t_WfMan  input_array_M=MWS.In.WfMan
  Model Source1 : Lib_Solve_ModelSource_TMATS/Model Source  T_vec_M=MWS.In.t_Alt  input_array_M=MWS.In.Alt
  Model Source10 : Lib_Solve_ModelSource_TMATS/Model Source  T_vec_M=MWS.In.t_PwrInLPOffNomMan  input_array_M=MWS.In.PwrInLPOffNomMan
  Model Source11 : Lib_Solve_ModelSource_TMATS/Model Source  T_vec_M=MWS.In.t_PwrInHPOffNomMan  input_array_M=MWS.In.PwrInHPOffNomMan
  Model Source12 : Lib_Solve_ModelSource_TMATS/Model Source  T_vec_M=MWS.In.t_PwrInHPEMOffNomMan  input_array_M=MWS.In.PwrInHPEMOffNomMan
  Model Source13 : Lib_Solve_ModelSource_TMATS/Model Source  T_vec_M=MWS.In.t_PwrInHPEMNomMan  input_array_M=MWS.In.PwrInHPEMNomMan
  Model Source14 : Lib_Solve_ModelSource_TMATS/Model Source  T_vec_M=MWS.In.t_PwrInLPEMOffNomMan  input_array_M=MWS.In.PwrInLPEMOffNomMan
  Model Source15 : Lib_Solve_ModelSource_TMATS/Model Source  T_vec_M=MWS.In.t_PwrInLPEMNomMan  input_array_M=MWS.In.PwrInLPEMNomMan
  Model Source16 : Lib_Solve_ModelSource_TMATS/Model Source  T_vec_M=MWS.In.t_PwrInSEMOffNomMan  input_array_M=MWS.In.PwrInSEMOffNomMan
  Model Source17 : Lib_Solve_ModelSource_TMATS/Model Source  T_vec_M=MWS.In.t_PwrInSEMNomMan  input_array_M=MWS.In.PwrInSEMNomMan
  Model Source18 : Lib_Solve_ModelSource_TMATS/Model Source  T_vec_M=MWS.In.t_PwrInREMOffNomMan  input_array_M=MWS.In.PwrInREMOffNomMan
  Model Source19 : Lib_Solve_ModelSource_TMATS/Model Source  T_vec_M=MWS.In.t_PwrInREMNomMan  input_array_M=MWS.In.PwrInREMNomMan
  Model Source2 : Lib_Solve_ModelSource_TMATS/Model Source  T_vec_M=MWS.In.t_dTamb  input_array_M=MWS.In.dTamb
  Model Source20 : Lib_Solve_ModelSource_TMATS/Model Source  T_vec_M=MWS.In.t_PwrInCEMOffNomMan  input_array_M=MWS.In.PwrInCEMOffNomMan
  Model Source21 : Lib_Solve_ModelSource_TMATS/Model Source  T_vec_M=MWS.In.t_PwrInCEMNomMan  input_array_M=MWS.In.PwrInCEMNomMan
  Model Source22 : Lib_Solve_ModelSource_TMATS/Model Source  T_vec_M=MWS.In.t_PwrInPEMOffNomMan  input_array_M=MWS.In.PwrInPEMOffNomMan
  Model Source23 : Lib_Solve_ModelSource_TMATS/Model Source  T_vec_M=MWS.In.t_PwrInPEMNomMan  input_array_M=MWS.In.PwrInPEMNomMan
  Model Source24 : Lib_Solve_ModelSource_TMATS/Model Source  T_vec_M=MWS.In.t_Boost  input_array_M=MWS.In.Boost
  Model Source25 : Lib_Solve_ModelSource_TMATS/Model Source  T_vec_M=MWS.In.t_EPT  input_array_M=MWS.In.EPT
  Model Source26 : Lib_Solve_ModelSource_TMATS/Model Source  T_vec_M=MWS.In.t_PExAC  input_array_M=MWS.In.PExAC
  Model Source27 : Lib_Solve_ModelSource_TMATS/Model Source  T_vec_M=MWS.In.t_Charge  input_array_M=MWS.In.Charge
  Model Source3 : Lib_Solve_ModelSource_TMATS/Model Source  T_vec_M=MWS.In.t_MN  input_array_M=MWS.In.MN
  Model Source4 : Lib_Solve_ModelSource_TMATS/Model Source  T_vec_M=MWS.In.t_PLA  input_array_M=MWS.In.PLA
  Model Source5 : Lib_Solve_ModelSource_TMATS/Model Source  T_vec_M=MWS.In.t_PwrInLPNomMan  input_array_M=MWS.In.PwrInLPNomMan
  Model Source6 : Lib_Solve_ModelSource_TMATS/Model Source  T_vec_M=MWS.In.t_VBVMan  input_array_M=MWS.In.VBVMan
  Model Source7 : Lib_Solve_ModelSource_TMATS/Model Source  T_vec_M=MWS.In.t_VAFNMan  input_array_M=MWS.In.VAFNMan
  Model Source8 : Lib_Solve_ModelSource_TMATS/Model Source  T_vec_M=MWS.In.t_N1cMan  input_array_M=MWS.In.N1cMan
  Model Source9 : Lib_Solve_ModelSource_TMATS/Model Source  T_vec_M=MWS.In.t_PwrInHPNomMan  input_array_M=MWS.In.PwrInHPNomMan
  SysInp : Outport
  wires:
  Model Source1/1 -> Bus Creator/1  "Alt"
  Model Source2/1 -> Bus Creator/2  "dT"
  Model Source3/1 -> Bus Creator/3  "MN"
  Bus Creator/1 -> Bus Creator2/1  "EngInp"
  Bus Creator5/1 -> Bus Creator2/2  "CntrlInp"
  Bus Creator2/1 -> SysInp/1  "SysInp"
  Model Source6/1 -> Bus Creator6/5  "VBVMan"
  Model Source7/1 -> Bus Creator6/7  "VAFNMan"
  Model Source4/1 -> Bus Creator1/1  "PLA"
  Bus Creator6/1 -> Bus Creator5/2  "ManualOp"
  Model Source/1 -> Bus Creator6/1  "WfMan"
  Constant1/1 -> Bus Creator6/2  "WfManEn"
  Constant4/1 -> Bus Creator6/8  "VAFNManEn"
  Constant3/1 -> Bus Creator6/6  "VBVManEn"
  Model Source8/1 -> Bus Creator6/3  "N1cMan"
  Constant5/1 -> Bus Creator6/4  "N1cManEn"
  Model Source5/1 -> Bus Creator6/9  "PwrInLPNomMan"
  Constant2/1 -> Bus Creator6/10  "PwrInLPNomManEn"
  Model Source10/1 -> Bus Creator6/11  "PwrInLPOffNomMan"
  Constant7/1 -> Bus Creator6/12  "PwrInLPOffNomManEn"
  Model Source9/1 -> Bus Creator6/13  "PwrInHPNomMan"
  Constant6/1 -> Bus Creator6/14  "PwrInHPNomManEn"
  Model Source11/1 -> Bus Creator6/15  "PwrInHPOffNomMan"
  Constant8/1 -> Bus Creator6/16  "PwrInHPOffNomManEn"
  Model Source15/1 -> Bus Creator6/17  "PwrInLPEMNomMan"
  Constant12/1 -> Bus Creator6/18  "PwrInLPEMNomManEn"
  Model Source14/1 -> Bus Creator6/19  "PwrInLPEMOffNomMan"
  Constant11/1 -> Bus Creator6/20  "PwrInLPEMOffNomManEn"
  Model Source13/1 -> Bus Creator6/21  "PwrInHPEMNomMan"
  Constant9/1 -> Bus Creator6/22  "PwrInHPEMNomManEn"
  Model Source12/1 -> Bus Creator6/23  "PwrInHPEMOffNomMan"
  Constant10/1 -> Bus Creator6/24  "PwrInHPEMOffNomManEn"
  Model Source17/1 -> Bus Creator6/25  "PwrInSEMNomMan"
  Constant14/1 -> Bus Creator6/26  "PwrInSEMNomManEn"
  Model Source16/1 -> Bus Creator6/27  "PwrInSEMOffNomMan"
  Constant13/1 -> Bus Creator6/28  "PwrInSEMOffNomManEn"
  Model Source19/1 -> Bus Creator6/29  "PwrInREMNomMan"
  Constant16/1 -> Bus Creator6/30  "PwrInREMNomManEn"
  Model Source18/1 -> Bus Creator6/31  "PwrInREMOffNomMan"
  Constant15/1 -> Bus Creator6/32  "PwrInREMOffNomManEn"
  Model Source21/1 -> Bus Creator6/33  "PwrInCEMNomMan"
  Constant18/1 -> Bus Creator6/34  "PwrInCEMNomManEn"
  Model Source20/1 -> Bus Creator6/35  "PwrInCEMOffNomMan"
  Constant17/1 -> Bus Creator6/36  "PwrInCEMOffNomManEn"
  Model Source23/1 -> Bus Creator6/37  "PwrInPEMNomMan"
  Constant20/1 -> Bus Creator6/38  "PwrInPEMNomManEn"
  Model Source22/1 -> Bus Creator6/39  "PwrInPEMOffNomMan"
  Constant19/1 -> Bus Creator6/40  "PwrInPEMOffNomManEn"
  Bus Creator1/1 -> Bus Creator5/1  "PilotCmd"
  Model Source24/1 -> Bus Creator1/2  "BoostToggle"
  Model Source25/1 -> Bus Creator1/3  "EPTToggle"
  Model Source26/1 -> Bus Creator/4  "PExAC"
  Model Source27/1 -> Bus Creator1/4  "ChargingToggle"

== system AGTF30SysDyn_PExPIn/Actuators/Carrier Electric Machine ==
  TrqEMCdmd : Inport
  NemC : Inport  Port=2
  Abs : Abs  SaturateOnIntegerOverflow=off
  Abs1 : Abs  SaturateOnIntegerOverflow=off
  Constant : Constant  Value=MWS.PowerSystem.EMC.PMax
  Constant1 : Constant  Value=MWS.In.Ts
  Constant2 : Constant  Value=MWS.Act.EMC.RLmax
  Constant3 : Constant  Value=MWS.Act.EMC.RLmin
  Divide : Product  Inputs=**
  Low Spool Electric Machine Dynamics : StateSpace  A=MWS.Act.EMC.A  B=MWS.Act.EMC.B  C=MWS.Act.EMC.C  D=MWS.Act.EMC.D  InitialCondition=MWS.Init.IC.TrqEMC
  Memory3 : Memory  InitialCondition=MWS.Init.IC.TrqEMC
  Memory5 : Memory  InitialCondition=MWS.Init.IC.NemC
  Power [hp] to Torque [ft-lb] : Subsystem
  Rate Limit Enforcement : MATLAB Function  TreatAsAtomicUnit=on
  Relational Operator : RelationalOperator  Operator=<=  OutDataTypeStr=boolean  RndMeth=Simplest  InputSameDT=off
  Saturation1 : Saturate  UpperLimit=MWS.PowerSystem.EMC.TrqMax  LowerLimit=-MWS.PowerSystem.EMC.TrqMax  LinearizeAsGain=off
  Sign : Signum
  Switch : Switch  Criteria=u2 > Threshold  SaturateOnIntegerOverflow=off  InputSameDT=off
  TrqEMCact : Outport  VectorParamsAs1DForOutWhenUnconnected=off
  wires:
  Low Spool Electric Machine Dynamics/1 -> Saturation1/1
  Constant/1 -> Power [hp] to Torque [ft-lb]/2(P)
  Saturation1/1 -> Switch/3, Sign/1, Abs/1
  Power [hp] to Torque [ft-lb]/1(Trq) -> Abs1/1
  Abs/1 -> Relational Operator/2
  Relational Operator/1 -> Switch/2
  Divide/1 -> Switch/1
  Sign/1 -> Divide/2
  Constant1/1 -> Rate Limit Enforcement/5(dt)
  Constant2/1 -> Rate Limit Enforcement/4(Mdot_hi)
  Constant3/1 -> Rate Limit Enforcement/3(Mdot_low)
  Memory3/1 -> Rate Limit Enforcement/2(M_old)
  Switch/1 -> Rate Limit Enforcement/1(M_preRL)
  NemC/1 -> Memory5/1
  Memory5/1 -> Power [hp] to Torque [ft-lb]/1(N)
  Rate Limit Enforcement/1(M_act) -> TrqEMCact/1, Memory3/1
  TrqEMCdmd/1 -> Low Spool Electric Machine Dynamics/1
  Abs1/1 -> Divide/1, Relational Operator/1

== system AGTF30SysDyn_PExPIn/Actuators/FMV ==
  Wfdmd : Inport
  1st order Actuator : Lib_Cntrl_FirstOrderActuator_TMATS/1st order Actuator  Gain_M=MWS.Act.FMV.Gain  Tau_M=MWS.Act.FMV.Tau  IC_M=MWS.Init.IC.Wf  MaxSat_M=MWS.Act.FMV.max  MinSat_M=MWS.Act.FMV.min  deadband_M=0.0  rateLimit_M=MWS.Act.FMV.rateLimit
  Wf delay : TransportDelay  DelayTime=MWS.Act.FMV.TWf_dly  InitialOutput=MWS.Init.IC.Wf
  Wfact : Outport
  wires:
  Wf delay/1 -> Wfact/1  "Wfact"
  Wfdmd/1 -> 1st order Actuator/1
  1st order Actuator/1 -> Wf delay/1

== system AGTF30SysDyn_PExPIn/Actuators/HPS Electric Machine ==
  TrqEMHdmd : Inport
  NemH : Inport  Port=2
  Abs : Abs  SaturateOnIntegerOverflow=off
  Abs1 : Abs  SaturateOnIntegerOverflow=off
  Constant : Constant  Value=MWS.PowerSystem.EMH.PMax
  Constant1 : Constant  Value=MWS.In.Ts
  Constant2 : Constant  Value=MWS.Act.EMH.RLmax
  Constant3 : Constant  Value=MWS.Act.EMH.RLmin
  Divide : Product  Inputs=**
  Low Spool Electric Machine Dynamics : StateSpace  A=MWS.Act.EMH.A  B=MWS.Act.EMH.B  C=MWS.Act.EMH.C  D=MWS.Act.EMH.D  InitialCondition=MWS.Init.IC.TrqEMH
  Memory3 : Memory  InitialCondition=MWS.Init.IC.TrqEMH
  Memory5 : Memory  InitialCondition=MWS.Init.IC.NemH
  Power [hp] to Torque [ft-lb] : Subsystem
  Rate Limit Enforcement : MATLAB Function  TreatAsAtomicUnit=on
  Relational Operator : RelationalOperator  Operator=<=  OutDataTypeStr=boolean  RndMeth=Simplest  InputSameDT=off
  Saturation1 : Saturate  UpperLimit=MWS.PowerSystem.EMH.TrqMax  LowerLimit=-MWS.PowerSystem.EMH.TrqMax  LinearizeAsGain=off
  Sign : Signum
  Switch : Switch  Criteria=u2 > Threshold  SaturateOnIntegerOverflow=off  InputSameDT=off
  TrqEMHact : Outport  VectorParamsAs1DForOutWhenUnconnected=off
  wires:
  Low Spool Electric Machine Dynamics/1 -> Saturation1/1
  Constant/1 -> Power [hp] to Torque [ft-lb]/2(P)
  Saturation1/1 -> Switch/3, Sign/1, Abs/1
  Power [hp] to Torque [ft-lb]/1(Trq) -> Abs1/1
  Abs/1 -> Relational Operator/2
  Relational Operator/1 -> Switch/2
  Divide/1 -> Switch/1
  Sign/1 -> Divide/2
  Constant1/1 -> Rate Limit Enforcement/5(dt)
  Constant2/1 -> Rate Limit Enforcement/4(Mdot_hi)
  Constant3/1 -> Rate Limit Enforcement/3(Mdot_low)
  Memory3/1 -> Rate Limit Enforcement/2(M_old)
  Switch/1 -> Rate Limit Enforcement/1(M_preRL)
  NemH/1 -> Memory5/1
  Memory5/1 -> Power [hp] to Torque [ft-lb]/1(N)
  Rate Limit Enforcement/1(M_act) -> TrqEMHact/1, Memory3/1
  TrqEMHdmd/1 -> Low Spool Electric Machine Dynamics/1
  Abs1/1 -> Divide/1, Relational Operator/1

== system AGTF30SysDyn_PExPIn/Actuators/LPS Electric Machine ==
  TrqEMLdmd : Inport
  NemL : Inport  Port=2
  Abs : Abs  SaturateOnIntegerOverflow=off
  Abs1 : Abs  SaturateOnIntegerOverflow=off
  Constant : Constant  Value=MWS.PowerSystem.EML.PMax
  Constant1 : Constant  Value=MWS.In.Ts
  Constant2 : Constant  Value=MWS.Act.EML.RLmax
  Constant3 : Constant  Value=MWS.Act.EML.RLmin
  Divide : Product  Inputs=**
  Low Spool Electric Machine Dynamics : StateSpace  A=MWS.Act.EML.A  B=MWS.Act.EML.B  C=MWS.Act.EML.C  D=MWS.Act.EML.D  InitialCondition=MWS.Init.IC.TrqEML
  Memory3 : Memory  InitialCondition=MWS.Init.IC.TrqEML
  Memory5 : Memory  InitialCondition=MWS.Init.IC.NemL
  Power [hp] to Torque [ft-lb] : Subsystem
  Rate Limit Enforcement : MATLAB Function  TreatAsAtomicUnit=on
  Relational Operator : RelationalOperator  Operator=<=  OutDataTypeStr=boolean  RndMeth=Simplest  InputSameDT=off
  Saturation1 : Saturate  UpperLimit=MWS.PowerSystem.EML.TrqMax  LowerLimit=-MWS.PowerSystem.EML.TrqMax  LinearizeAsGain=off
  Sign : Signum
  Switch : Switch  Criteria=u2 > Threshold  SaturateOnIntegerOverflow=off  InputSameDT=off
  TrqEMLact : Outport  VectorParamsAs1DForOutWhenUnconnected=off
  wires:
  Low Spool Electric Machine Dynamics/1 -> Saturation1/1
  Constant/1 -> Power [hp] to Torque [ft-lb]/2(P)
  Saturation1/1 -> Switch/3, Sign/1, Abs/1
  Power [hp] to Torque [ft-lb]/1(Trq) -> Abs1/1
  Abs/1 -> Relational Operator/2
  Relational Operator/1 -> Switch/2
  Divide/1 -> Switch/1
  Sign/1 -> Divide/2
  Constant1/1 -> Rate Limit Enforcement/5(dt)
  Constant2/1 -> Rate Limit Enforcement/4(Mdot_hi)
  Constant3/1 -> Rate Limit Enforcement/3(Mdot_low)
  Memory3/1 -> Rate Limit Enforcement/2(M_old)
  Switch/1 -> Rate Limit Enforcement/1(M_preRL)
  NemL/1 -> Memory5/1
  Memory5/1 -> Power [hp] to Torque [ft-lb]/1(N)
  Rate Limit Enforcement/1(M_act) -> TrqEMLact/1, Memory3/1
  TrqEMLdmd/1 -> Low Spool Electric Machine Dynamics/1
  Abs1/1 -> Divide/1, Relational Operator/1

== system AGTF30SysDyn_PExPIn/Actuators/Planet Gear Electric Machine ==
  TrqEMPdmd : Inport
  NemP : Inport  Port=2
  Abs : Abs  SaturateOnIntegerOverflow=off
  Abs1 : Abs  SaturateOnIntegerOverflow=off
  Constant : Constant  Value=MWS.PowerSystem.EMP.PMax
  Constant1 : Constant  Value=MWS.In.Ts
  Constant2 : Constant  Value=MWS.Act.EMP.RLmax
  Constant3 : Constant  Value=MWS.Act.EMP.RLmin
  Divide : Product  Inputs=**
  Low Spool Electric Machine Dynamics : StateSpace  A=MWS.Act.EMP.A  B=MWS.Act.EMP.B  C=MWS.Act.EMP.C  D=MWS.Act.EMP.D  InitialCondition=MWS.Init.IC.TrqEMP
  Memory3 : Memory  InitialCondition=MWS.Init.IC.TrqEMP
  Memory5 : Memory  InitialCondition=MWS.Init.IC.NemP
  Power [hp] to Torque [ft-lb] : Subsystem
  Rate Limit Enforcement : MATLAB Function  TreatAsAtomicUnit=on
  Relational Operator : RelationalOperator  Operator=<=  OutDataTypeStr=boolean  RndMeth=Simplest  InputSameDT=off
  Saturation1 : Saturate  UpperLimit=MWS.PowerSystem.EMP.TrqMax  LowerLimit=-MWS.PowerSystem.EMP.TrqMax  LinearizeAsGain=off
  Sign : Signum
  Switch : Switch  Criteria=u2 > Threshold  SaturateOnIntegerOverflow=off  InputSameDT=off
  TrqEMPact : Outport  VectorParamsAs1DForOutWhenUnconnected=off
  wires:
  Low Spool Electric Machine Dynamics/1 -> Saturation1/1
  Constant/1 -> Power [hp] to Torque [ft-lb]/2(P)
  Saturation1/1 -> Switch/3, Sign/1, Abs/1
  Power [hp] to Torque [ft-lb]/1(Trq) -> Abs1/1
  Abs/1 -> Relational Operator/2
  Relational Operator/1 -> Switch/2
  Divide/1 -> Switch/1
  Sign/1 -> Divide/2
  Constant1/1 -> Rate Limit Enforcement/5(dt)
  Constant2/1 -> Rate Limit Enforcement/4(Mdot_hi)
  Constant3/1 -> Rate Limit Enforcement/3(Mdot_low)
  Memory3/1 -> Rate Limit Enforcement/2(M_old)
  Switch/1 -> Rate Limit Enforcement/1(M_preRL)
  NemP/1 -> Memory5/1
  Memory5/1 -> Power [hp] to Torque [ft-lb]/1(N)
  Rate Limit Enforcement/1(M_act) -> TrqEMPact/1, Memory3/1
  TrqEMPdmd/1 -> Low Spool Electric Machine Dynamics/1
  Abs1/1 -> Divide/1, Relational Operator/1

== system AGTF30SysDyn_PExPIn/Actuators/Ring Gear Electric Machine ==
  TrqEMRdmd : Inport
  NemR : Inport  Port=2
  Abs : Abs  SaturateOnIntegerOverflow=off
  Abs1 : Abs  SaturateOnIntegerOverflow=off
  Constant : Constant  Value=MWS.PowerSystem.EMR.PMax
  Constant1 : Constant  Value=MWS.In.Ts
  Constant2 : Constant  Value=MWS.Act.EMR.RLmax
  Constant3 : Constant  Value=MWS.Act.EMR.RLmin
  Divide : Product  Inputs=**
  Low Spool Electric Machine Dynamics : StateSpace  A=MWS.Act.EMR.A  B=MWS.Act.EMR.B  C=MWS.Act.EMR.C  D=MWS.Act.EMR.D  InitialCondition=MWS.Init.IC.TrqEMR
  Memory3 : Memory  InitialCondition=MWS.Init.IC.TrqEMR
  Memory5 : Memory  InitialCondition=MWS.Init.IC.NemR
  Power [hp] to Torque [ft-lb] : Subsystem
  Rate Limit Enforcement : MATLAB Function  TreatAsAtomicUnit=on
  Relational Operator : RelationalOperator  Operator=<=  OutDataTypeStr=boolean  RndMeth=Simplest  InputSameDT=off
  Saturation1 : Saturate  UpperLimit=MWS.PowerSystem.EMR.TrqMax  LowerLimit=-MWS.PowerSystem.EMR.TrqMax  LinearizeAsGain=off
  Sign : Signum
  Switch : Switch  Criteria=u2 > Threshold  SaturateOnIntegerOverflow=off  InputSameDT=off
  TrqEMRact : Outport  VectorParamsAs1DForOutWhenUnconnected=off
  wires:
  Low Spool Electric Machine Dynamics/1 -> Saturation1/1
  Constant/1 -> Power [hp] to Torque [ft-lb]/2(P)
  Saturation1/1 -> Switch/3, Sign/1, Abs/1
  Power [hp] to Torque [ft-lb]/1(Trq) -> Abs1/1
  Abs/1 -> Relational Operator/2
  Relational Operator/1 -> Switch/2
  Divide/1 -> Switch/1
  Sign/1 -> Divide/2
  Constant1/1 -> Rate Limit Enforcement/5(dt)
  Constant2/1 -> Rate Limit Enforcement/4(Mdot_hi)
  Constant3/1 -> Rate Limit Enforcement/3(Mdot_low)
  Memory3/1 -> Rate Limit Enforcement/2(M_old)
  Switch/1 -> Rate Limit Enforcement/1(M_preRL)
  NemR/1 -> Memory5/1
  Memory5/1 -> Power [hp] to Torque [ft-lb]/1(N)
  Rate Limit Enforcement/1(M_act) -> TrqEMRact/1, Memory3/1
  TrqEMRdmd/1 -> Low Spool Electric Machine Dynamics/1
  Abs1/1 -> Divide/1, Relational Operator/1

== system AGTF30SysDyn_PExPIn/Actuators/Sun Gear Electric Machine ==
  TrqEMSdmd : Inport
  NemS : Inport  Port=2
  Abs : Abs  SaturateOnIntegerOverflow=off
  Abs1 : Abs  SaturateOnIntegerOverflow=off
  Constant : Constant  Value=MWS.PowerSystem.EMS.PMax
  Constant1 : Constant  Value=MWS.In.Ts
  Constant2 : Constant  Value=MWS.Act.EMS.RLmax
  Constant3 : Constant  Value=MWS.Act.EMS.RLmin
  Divide : Product  Inputs=**
  Low Spool Electric Machine Dynamics : StateSpace  A=MWS.Act.EMS.A  B=MWS.Act.EMS.B  C=MWS.Act.EMS.C  D=MWS.Act.EMS.D  InitialCondition=MWS.Init.IC.TrqEMS
  Memory3 : Memory  InitialCondition=MWS.Init.IC.TrqEMS
  Memory5 : Memory  InitialCondition=MWS.Init.IC.NemS
  Power [hp] to Torque [ft-lb] : Subsystem
  Rate Limit Enforcement : MATLAB Function  TreatAsAtomicUnit=on
  Relational Operator : RelationalOperator  Operator=<=  OutDataTypeStr=boolean  RndMeth=Simplest  InputSameDT=off
  Saturation1 : Saturate  UpperLimit=MWS.PowerSystem.EMS.TrqMax  LowerLimit=-MWS.PowerSystem.EMS.TrqMax  LinearizeAsGain=off
  Sign : Signum
  Switch : Switch  Criteria=u2 > Threshold  SaturateOnIntegerOverflow=off  InputSameDT=off
  TrqEMSact : Outport  VectorParamsAs1DForOutWhenUnconnected=off
  wires:
  Low Spool Electric Machine Dynamics/1 -> Saturation1/1
  Constant/1 -> Power [hp] to Torque [ft-lb]/2(P)
  Saturation1/1 -> Switch/3, Sign/1, Abs/1
  Power [hp] to Torque [ft-lb]/1(Trq) -> Abs1/1
  Abs/1 -> Relational Operator/2
  Relational Operator/1 -> Switch/2
  Divide/1 -> Switch/1
  Sign/1 -> Divide/2
  Constant1/1 -> Rate Limit Enforcement/5(dt)
  Constant2/1 -> Rate Limit Enforcement/4(Mdot_hi)
  Constant3/1 -> Rate Limit Enforcement/3(Mdot_low)
  Memory3/1 -> Rate Limit Enforcement/2(M_old)
  Switch/1 -> Rate Limit Enforcement/1(M_preRL)
  NemS/1 -> Memory5/1
  Memory5/1 -> Power [hp] to Torque [ft-lb]/1(N)
  Rate Limit Enforcement/1(M_act) -> TrqEMSact/1, Memory3/1
  TrqEMSdmd/1 -> Low Spool Electric Machine Dynamics/1
  Abs1/1 -> Divide/1, Relational Operator/1

== system AGTF30SysDyn_PExPIn/Actuators/VAFN ==
  VAFNdmd : Inport
  Saturation1 : Saturate  UpperLimit=MWS.Act.VAFN_max  LowerLimit=0  LinearizeAsGain=off
  VAFN Dynamics : StateSpace  A=MWS.Act.VAFN.A  B=MWS.Act.VAFN.B  C=MWS.Act.VAFN.C  D=MWS.Act.VAFN.D  InitialCondition=MWS.Init.IC.VAFN
  VAFNact : Outport
  wires:
  Saturation1/1 -> VAFNact/1
  VAFNdmd/1 -> VAFN Dynamics/1
  VAFN Dynamics/1 -> Saturation1/1

== system AGTF30SysDyn_PExPIn/Actuators/VBV ==
  VBVdmd : Inport
  1st order Actuator : Lib_Cntrl_FirstOrderActuator_TMATS/1st order Actuator  Gain_M=MWS.Act.VBV.Gain  Tau_M=MWS.Act.VBV.Tau  IC_M=MWS.Init.IC.VBV  MaxSat_M=MWS.Act.VBV.max  MinSat_M=MWS.Act.VBV.min  deadband_M=0.0  rateLimit_M=100000
  VBVact : Outport
  wires:
  VBVdmd/1 -> 1st order Actuator/1
  1st order Actuator/1 -> VBVact/1  "VBVact"
